simulink model "early_return_logic_eg1"  (R2018a)
settings: Solver=VariableStepAuto  StartTime=0.0  StopTime=10.0  RelTol=1e-3
settings Model: Creator=86188  LastModifiedBy=86188

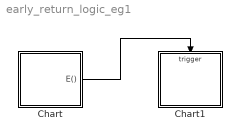
== system early_return_logic_eg1 ==
  Chart : Stateflow chart  TreatAsAtomicUnit=on
  Chart1 : Stateflow chart  TreatAsAtomicUnit=on
  wires:
  Chart/1(E()) -> Chart1/Trigger

== stateflow chart early_return_logic_eg1/Chart1 ==
  settings: executeAtInitialization=1
  state A
    en:[y,x]=enA();
    du:duA();
    ex:exA();
  state B
    en:enB();
    du:duB();
    ex:exA();
  state C
    en:enC();
    du:duC();
    ex:exC();
  (default) -> A
  A -> B [order 1] : E{condition();send(F)}
  A -> C [order 2] : F
  data: x function_output; y function_output
  events: E input FUNCTION_CALL_EVENT; F local FUNCTION_CALL_EVENT
  function exA:
    | function exA
    | fprintf("exA is executing ");
  function [x,y]=enA:
    | function [x,y]=enA()
    | x=0;
    | x=x+1;
    | y=4;
    | fprintf("enA is executing "+x);
  function duA:
    | function duA
    | fprintf("duA is executing ");
  function duB:
    | function duB
    | fprintf("duB is executing ");
  function exB:
    | function exB
    | fprintf("exB is executing ");
  function enB:
    | function enB
    | fprintf("enB is executing ");
  function condition:
    | function condition
    | fprintf("condition action is executing ");
  function enC:
    | function enC
    | fprintf("enC is executing ");
  function duC:
    | function duC
    | fprintf("duC is executing ");
  function exC:
    | function exC
    | fprintf("exC is executing ");

== stateflow chart early_return_logic_eg1/Chart ==
  state A
    send(E)
  (default) -> A
  events: E output FUNCTION_CALL_EVENT
